simulink model "AutoDRIVE"  (R2024b)
settings: Solver=VariableStepAuto  StartTime=0.0  StopTime=10.0  RelTol=1e-3
undefined symbols (not defined in the file): gray, robotGoal
settings Model: DataDictionary=DataDictionary.sldd  Creator=jkcolem  LastModifiedBy=tsamak
settings SFSimCC: SimTargetLang=C++

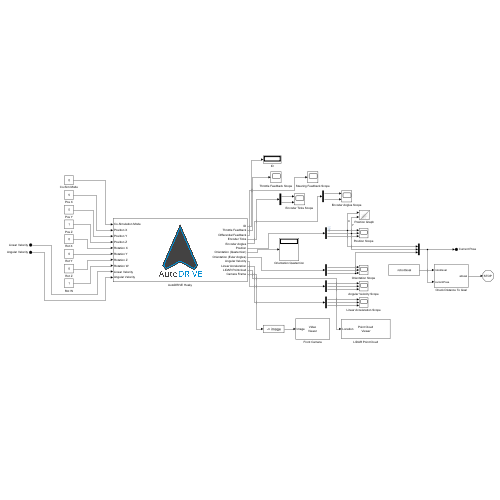
[thumbnail: Simulink's stored preview of the top-level diagram]
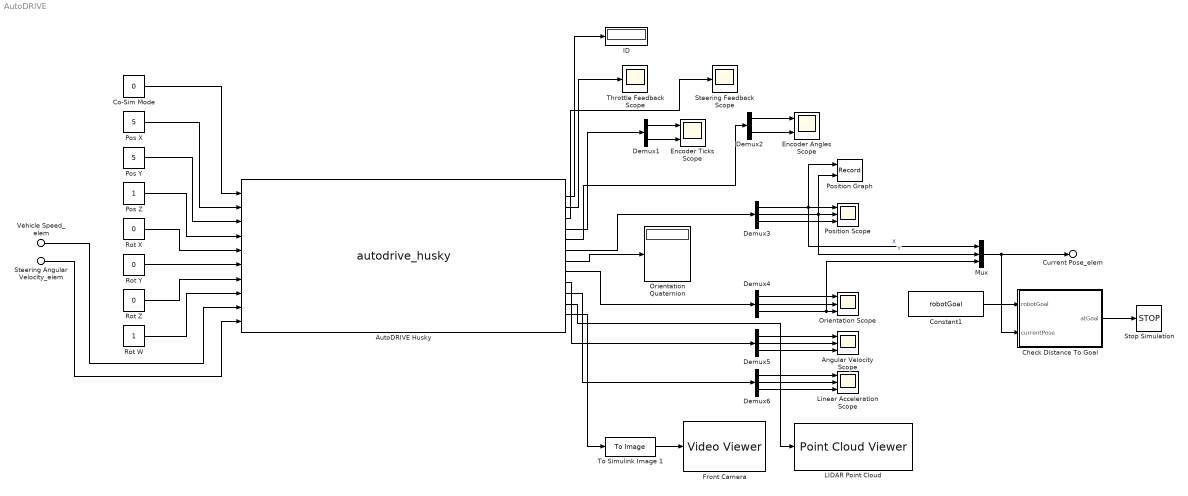
== system AutoDRIVE ==
  Vehicle Speed_elem : Inport  PortName=Linear Velocity
  Steering Angular Velocity_elem : Inport  Port=2  PortName=Angular Velocity
  Angular Velocity Scope : Scope  NumInputPorts=3
  AutoDRIVE Husky : M-S-Function  FunctionName=autodrive_husky  Parameters=Port  mask{Port=4567}
      mask Display:
      | image('autodrive_logo.png');
      | port_label('input', 1, 'Co-Simulation Mode');
      | port_label('input', 2, 'Position X');
      | port_label('input', 3, 'Position Y');
      | port_label('input', 4, 'Position Z');
      | port_label('input', 5, 'Rotation X');
      | port_label('input', 6, 'Rotation Y');
      | port_label('input', 7, 'Rotation Z');
      | port_label('input', 8, 'Rotation W');
      | port_label('input', 9, 'Linear Velocity');
      | port_label('input', 10, 'Angular Velocity');
      | port_label('output', 1, 'ID');
      | port_label('output', 2, 'Throttle Feedback');
      | port_label('output', 3, 'Differential Feedback');
      | port_label('output', 4, 'Encoder Ticks');
      | port_label('output', 5, 'Encoder Angles');
      | port_label('output', 6, 'Position');
      | port_label('output', 7, 'Orientation (Quaternion)');
      | port_label('output', 8, 'Orientation (Euler Angles)');
      | port_label('output', 9, 'Angular Velocity');
      | port_label('output', 10, 'Linear Acceleration');
      | port_label('output', 11, 'LIDAR Pointcloud');
      | port_label('output', 12, 'Camera Frame');
  Check Distance To Goal : Subsystem
  Co-Sim Mode : Constant  Value=0  OutDataTypeStr=uint8
  Constant1 : Constant  Value=robotGoal
  Demux1 : Demux  Outputs=2
  Demux2 : Demux  Outputs=2
  Demux{3..6} (4 alike) : Demux  Outputs=3
  Encoder Angles Scope : Scope  NumInputPorts=2
  Encoder Ticks Scope : Scope  NumInputPorts=2
  Front Camera : VideoViewer  colormapValue=gray(256)  FigPos=[1236.33333333333 936 470 287.333333333333]
  ID : Display
  LIDAR Point Cloud : PointCloudViewer  FigPos=[1235.66666666667 541.333333333333 469.333333333333 301.333333333333]
  Linear Acceleration Scope : Scope  NumInputPorts=3
  Mux : Mux  Inputs=3
  Orientation Quaternion : Display
  Orientation Scope : Scope  NumInputPorts=3
  Pos X : Constant  Value=5
  Pos Y : Constant  Value=5
  Pos Z : Constant
  Position Graph : Record  FileSettingsInternal="{\"entries\":[{\"content\":{\"excelSettings\":{\"content\":{},\"type\":\"Streamout.ExcelSettings\"}},\"type\":\"Streamout.FileSettingStorage\",\"uuid\":\"\"}],\"packageUris\":[\"http:\\/\\/schema.mathworks.com\\/mf0\\/streamout_blocks\\/R2020a\"],\"version\":\"1.0\"}"  Layout=[1 1]  SignalsInternal="{\"entries\":[{\"content\":{\"signals\":[{\"content\":{\"blockPath\":[],\"dimensions\":[1,1],\"domain\":\"\",\"lineColor\":\"#0072bd\",\"lineWidth\":2,\"port\":1,\"signalID\":1,\"signalName\":\"X\"},\"type\":\"RecordBlkView.Signal\",\"uuid\":\"\"},{\"content\":{\"blockPath\":[],\"dimensions\":[1,1],\"domain\":\"\",\"lineColor\":\"#d95319\",\"lineWidth\":2,\"port\":2,\"signalID\":2,\"signalName\":\"Y\"},\"type\":\"RecordBlkView.Signal\",\"uuid\":\"\"}]},\"type\":\"RecordBlkView.InputSignals\",\"uuid\":\"\"}],\"packageUris\":[\"http:\\/\\/schema.mathworks.com\\/mf0\\/streamout_blocks\\/R2020a\"],\"version\":\"1.0\"}"  VisualizationBindings="{\"xyplotplugin\":{\"info\":[{\"series\":[],\"subplotID\":1}]}}"  CompatibilityTag=XY
  Position Scope : Scope  NumInputPorts=3
  Rot W : Constant
  Rot X : Constant  Value=0
  Rot Y : Constant  Value=0
  Rot Z : Constant  Value=0
  Steering Feedback Scope : Scope
  Stop Simulation : Stop
  Throttle Feedback Scope : Scope
  To Simulink Image 1 : ToImage
  Current Pose_elem : Outport  PortName=Current Pose
  wires:
  Co-Sim Mode/1 -> AutoDRIVE Husky/1
  AutoDRIVE Husky/1 -> ID/1
  Pos X/1 -> AutoDRIVE Husky/2
  Demux4/1 -> Orientation Scope/1
  Rot Y/1 -> AutoDRIVE Husky/6
  Demux4/3 -> Mux/3, Orientation Scope/3
  Demux1/1 -> Encoder Ticks Scope/1
  AutoDRIVE Husky/12 -> To Simulink Image 1/1
  Steering Angular Velocity_elem/1 -> AutoDRIVE Husky/10
  Rot W/1 -> AutoDRIVE Husky/8
  Demux1/2 -> Encoder Ticks Scope/2
  Pos Z/1 -> AutoDRIVE Husky/4
  AutoDRIVE Husky/4 -> Demux1/1
  Demux2/2 -> Encoder Angles Scope/2
  Pos Y/1 -> AutoDRIVE Husky/3
  Rot Z/1 -> AutoDRIVE Husky/7
  Demux5/2 -> Angular Velocity Scope/2
  To Simulink Image 1/1 -> Front Camera/1
  AutoDRIVE Husky/7 -> Orientation Quaternion/1
  Rot X/1 -> AutoDRIVE Husky/5
  AutoDRIVE Husky/3 -> Steering Feedback Scope/1
  Demux3/3 -> Position Scope/3
  Demux6/3 -> Linear Acceleration Scope/3
  Demux3/2 -> Mux/2, Position Scope/2, Position Graph/2  "Y"
  Demux4/2 -> Orientation Scope/2
  Demux6/2 -> Linear Acceleration Scope/2
  AutoDRIVE Husky/9 -> Demux5/1
  AutoDRIVE Husky/11 -> LIDAR Point Cloud/1
  Demux3/1 -> Mux/1, Position Scope/1, Position Graph/1  "X"
  AutoDRIVE Husky/8 -> Demux4/1
  AutoDRIVE Husky/6 -> Demux3/1
  Demux2/1 -> Encoder Angles Scope/1
  Demux5/1 -> Angular Velocity Scope/1
  AutoDRIVE Husky/10 -> Demux6/1
  AutoDRIVE Husky/5 -> Demux2/1
  AutoDRIVE Husky/2 -> Throttle Feedback Scope/1
  Demux6/1 -> Linear Acceleration Scope/1
  Vehicle Speed_elem/1 -> AutoDRIVE Husky/9
  Demux5/3 -> Angular Velocity Scope/3
  Mux/1 -> Current Pose_elem/1, Check Distance To Goal/2(currentPose)
  Check Distance To Goal/1(atGoal) -> Stop Simulation/1
  Constant1/1 -> Check Distance To Goal/1(robotGoal)

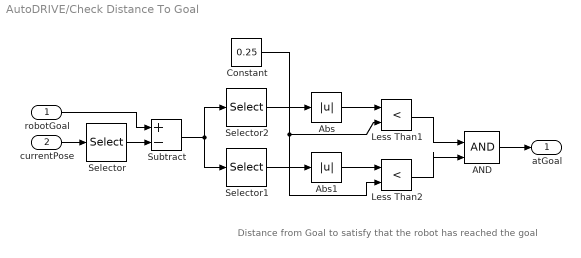
== system AutoDRIVE/Check Distance To Goal ==
  note: Distance from Goal to satisfy that the robot has reached the goal
  robotGoal : Inport
  currentPose : Inport  Port=2
  AND : Logic  IconShape=distinctive  AllPortsSameDT=off  OutDataTypeStr=boolean
  Abs : Abs  SaturateOnIntegerOverflow=off
  Abs1 : Abs  SaturateOnIntegerOverflow=off
  Constant : Constant  Value=0.25
  Less Than1 : RelationalOperator  Operator=<  OutDataTypeStr=boolean  RndMeth=Simplest  InputSameDT=off
  Less Than2 : RelationalOperator  Operator=<  OutDataTypeStr=boolean  RndMeth=Simplest  InputSameDT=off
  Selector : Selector  InputPortWidth=3  IndexOptions=Index vector (dialog)  Indices=[1 2]  OutputSizes=1
  Selector1 : Selector  InputPortWidth=2  IndexOptions=Index vector (dialog)  Indices=[2]  OutputSizes=1
  Selector2 : Selector  InputPortWidth=2  IndexOptions=Index vector (dialog)  Indices=[1]  OutputSizes=1
  Subtract : Sum  Inputs=+-
  atGoal : Outport
  wires:
  robotGoal/1 -> Subtract/1
  Subtract/1 -> Selector2/1, Selector1/1
  Selector/1 -> Subtract/2
  currentPose/1 -> Selector/1
  Constant/1 -> Less Than2/2, Less Than1/2
  AND/1 -> atGoal/1
  Selector1/1 -> Abs1/1
  Abs1/1 -> Less Than2/1
  Selector2/1 -> Abs/1
  Abs/1 -> Less Than1/1
  Less Than1/1 -> AND/1
  Less Than2/1 -> AND/2
